simulink model "Flex_simulink"  (R2018a)
settings: Solver=FixedStepDiscrete  StartTime=0.0  StopTime=inf  FixedStep=0.00005  RelTol=1e-3  EnableMultiTasking=on
PreLoadFcn:
  | Ts = 0.001;
InitFcn:
  | Ts = 0.001;
values from neighbouring files (symbols this model uses):
  I_limit = 500    [init.m]
libraries: xpcethercatlib x91, simulink x54, slrtlib x2
(part 2 of 2)

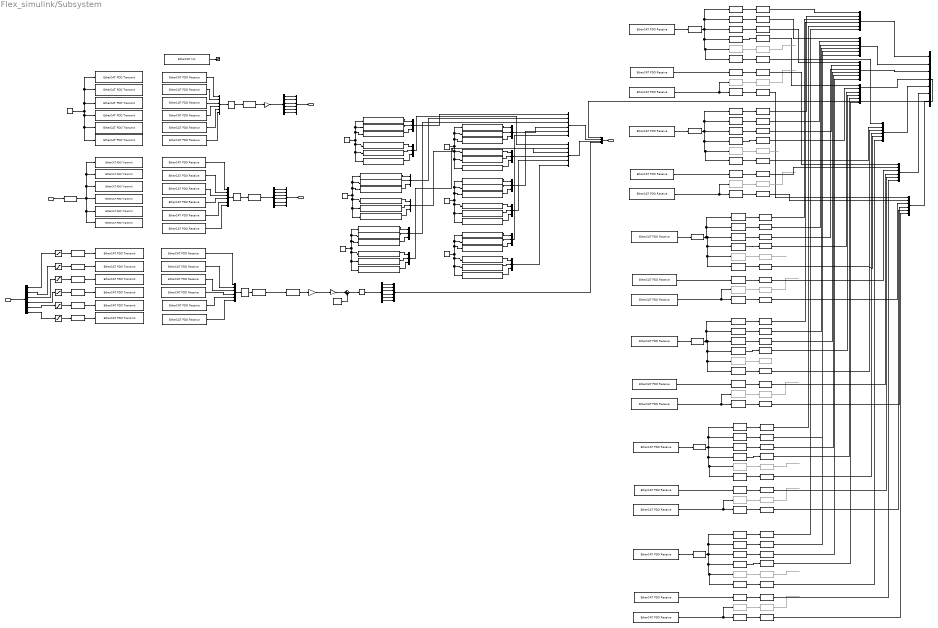
== system Flex_simulink/Subsystem ==
  Current [mA] : Inport
  Control word : Inport  Port=2
  Analog output voltage : Constant  Value=10000  OutDataTypeStr=int16
  Bus Creator{,2,4..8,20..21,23..28} (15 alike) : BusCreator  Inputs=6
  Bus Creator{1,3,10..19} (12 alike) : BusCreator  Inputs=3
  Bus Creator22 : BusCreator  Inputs=7
  Bus Creator9 : BusCreator  Inputs=4
  Bus Selector : BusSelector  OutputSignals=signal1,signal2,signal3,signal4,signal5,signal6
  Bus to Vector : BusToVector
  Bus to Vector1 : BusToVector
  Bus to Vector2 : BusToVector
  Constant : Constant  Value=-225
  Constant{1..6} (6 alike) : Constant  OutDataTypeStr=int32  SampleTime=1
  Data Type Conversion : DataTypeConversion  OutDataTypeStr=double
  Data Type Conversion1 : DataTypeConversion  OutDataTypeStr=double
  Data Type Conversion{3,10,21,27,31,37,41,47,51,57,61,67} (12 alike) : DataTypeConversion  Commented=on  OutDataTypeStr=boolean
  Data Type Conversion{2,6,8,11..14,22..26,28,30,32..36,38,40,42..46,48,50,52..56,58,60,62..66,68,70} (42 alike) : DataTypeConversion  OutDataTypeStr=boolean
  Data Type Conversion{4,9,15,17..20} (7 alike) : DataTypeConversion  OutDataTypeStr=int32
  Data Type Conversion16 : DataTypeConversion  OutDataTypeStr=uint16
  Data Type Conversion{7,29,39,49,59,69} (6 alike) : DataTypeConversion  OutDataTypeStr=uint16  RndMeth=Round
  Data Type Conversion5 : DataTypeConversion  OutDataTypeStr=double
  Demux : Demux  Outputs=6
  Demux1 : Demux  Outputs=6
  Demux2 : Demux  Outputs=6
  EtherCAT Async SDO Upload : xpcethercatlib/EtherCAT Async SDO Upload  index=8192  subIndex=1  sig_type=uint32  sig_dim=1  device_id=0  slave_name=Drive 2 (AKD)  sample_time=1  slave_addr=1001  selected_slave=Term 1 (EK1100)  timeout=500  slave_found=1
      settings: SourceProductName=Simulink Real-Time  SourceProductBaseCode=XP
  EtherCAT Async SDO Upload1 : xpcethercatlib/EtherCAT Async SDO Upload  index=8192  subIndex=2  sig_type=uint32  sig_dim=1  device_id=0  slave_name=Drive 2 (AKD)  sample_time=1  slave_addr=1001  selected_slave=Term 1 (EK1100)  timeout=500  slave_found=1
      settings: SourceProductName=Simulink Real-Time  SourceProductBaseCode=XP
  EtherCAT Async SDO Upload10 : xpcethercatlib/EtherCAT Async SDO Upload  index=8193  subIndex=2  sig_type=uint32  sig_dim=1  device_id=0  slave_name=Drive 3 (AKD)  sample_time=1  slave_addr=1002  selected_slave=Term 1 (EK1100)  timeout=500  slave_found=1
      settings: SourceProductName=Simulink Real-Time  SourceProductBaseCode=XP
  EtherCAT Async SDO Upload11 : xpcethercatlib/EtherCAT Async SDO Upload  index=8193  subIndex=3  sig_type=uint32  sig_dim=1  device_id=0  slave_name=Drive 3 (AKD)  sample_time=1  slave_addr=1002  selected_slave=Term 1 (EK1100)  timeout=500  slave_found=1
      settings: SourceProductName=Simulink Real-Time  SourceProductBaseCode=XP
  EtherCAT Async SDO Upload12 : xpcethercatlib/EtherCAT Async SDO Upload  index=8192  subIndex=1  sig_type=uint32  sig_dim=1  device_id=0  slave_name=Drive 4 (AKD)  sample_time=1  slave_addr=1003  selected_slave=Term 1 (EK1100)  timeout=500  slave_found=1
      settings: SourceProductName=Simulink Real-Time  SourceProductBaseCode=XP
  EtherCAT Async SDO Upload13 : xpcethercatlib/EtherCAT Async SDO Upload  index=8192  subIndex=2  sig_type=uint32  sig_dim=1  device_id=0  slave_name=Drive 4 (AKD)  sample_time=1  slave_addr=1003  selected_slave=Term 1 (EK1100)  timeout=500  slave_found=1
      settings: SourceProductName=Simulink Real-Time  SourceProductBaseCode=XP
  EtherCAT Async SDO Upload14 : xpcethercatlib/EtherCAT Async SDO Upload  index=8192  subIndex=3  sig_type=uint32  sig_dim=1  device_id=0  slave_name=Drive 4 (AKD)  sample_time=1  slave_addr=1003  selected_slave=Term 1 (EK1100)  timeout=500  slave_found=1
      settings: SourceProductName=Simulink Real-Time  SourceProductBaseCode=XP
  EtherCAT Async SDO Upload15 : xpcethercatlib/EtherCAT Async SDO Upload  index=8193  subIndex=1  sig_type=uint32  sig_dim=1  device_id=0  slave_name=Drive 4 (AKD)  sample_time=1  slave_addr=1003  selected_slave=Term 1 (EK1100)  timeout=500  slave_found=1
      settings: SourceProductName=Simulink Real-Time  SourceProductBaseCode=XP
  EtherCAT Async SDO Upload16 : xpcethercatlib/EtherCAT Async SDO Upload  index=8193  subIndex=2  sig_type=uint32  sig_dim=1  device_id=0  slave_name=Drive 4 (AKD)  sample_time=1  slave_addr=1003  selected_slave=Term 1 (EK1100)  timeout=500  slave_found=1
      settings: SourceProductName=Simulink Real-Time  SourceProductBaseCode=XP
  EtherCAT Async SDO Upload17 : xpcethercatlib/EtherCAT Async SDO Upload  index=8193  subIndex=3  sig_type=uint32  sig_dim=1  device_id=0  slave_name=Drive 4 (AKD)  sample_time=1  slave_addr=1003  selected_slave=Term 1 (EK1100)  timeout=500  slave_found=1
      settings: SourceProductName=Simulink Real-Time  SourceProductBaseCode=XP
  EtherCAT Async SDO Upload18 : xpcethercatlib/EtherCAT Async SDO Upload  index=8192  subIndex=1  sig_type=uint32  sig_dim=1  device_id=0  slave_name=Drive 5 (AKD)  sample_time=1  slave_addr=1004  selected_slave=Term 1 (EK1100)  timeout=500  slave_found=1
      settings: SourceProductName=Simulink Real-Time  SourceProductBaseCode=XP
  EtherCAT Async SDO Upload19 : xpcethercatlib/EtherCAT Async SDO Upload  index=8192  subIndex=2  sig_type=uint32  sig_dim=1  device_id=0  slave_name=Drive 5 (AKD)  sample_time=1  slave_addr=1004  selected_slave=Term 1 (EK1100)  timeout=500  slave_found=1
      settings: SourceProductName=Simulink Real-Time  SourceProductBaseCode=XP
  EtherCAT Async SDO Upload2 : xpcethercatlib/EtherCAT Async SDO Upload  index=8192  subIndex=3  sig_type=uint32  sig_dim=1  device_id=0  slave_name=Drive 1 (AKD)  sample_time=1  slave_addr=1001  selected_slave=Term 1 (EK1100)  timeout=500  slave_found=1
      settings: SourceProductName=Simulink Real-Time  SourceProductBaseCode=XP
  EtherCAT Async SDO Upload20 : xpcethercatlib/EtherCAT Async SDO Upload  index=8192  subIndex=3  sig_type=uint32  sig_dim=1  device_id=0  slave_name=Drive 5 (AKD)  sample_time=1  slave_addr=1004  selected_slave=Term 1 (EK1100)  timeout=500  slave_found=1
      settings: SourceProductName=Simulink Real-Time  SourceProductBaseCode=XP
  EtherCAT Async SDO Upload21 : xpcethercatlib/EtherCAT Async SDO Upload  index=8193  subIndex=1  sig_type=uint32  sig_dim=1  device_id=0  slave_name=Drive 5 (AKD)  sample_time=1  slave_addr=1004  selected_slave=Term 1 (EK1100)  timeout=500  slave_found=1
      settings: SourceProductName=Simulink Real-Time  SourceProductBaseCode=XP
  EtherCAT Async SDO Upload22 : xpcethercatlib/EtherCAT Async SDO Upload  index=8193  subIndex=2  sig_type=uint32  sig_dim=1  device_id=0  slave_name=Drive 5 (AKD)  sample_time=1  slave_addr=1004  selected_slave=Term 1 (EK1100)  timeout=500  slave_found=1
      settings: SourceProductName=Simulink Real-Time  SourceProductBaseCode=XP
  EtherCAT Async SDO Upload23 : xpcethercatlib/EtherCAT Async SDO Upload  index=8193  subIndex=3  sig_type=uint32  sig_dim=1  device_id=0  slave_name=Drive 5 (AKD)  sample_time=1  slave_addr=1004  selected_slave=Term 1 (EK1100)  timeout=500  slave_found=1
      settings: SourceProductName=Simulink Real-Time  SourceProductBaseCode=XP
  EtherCAT Async SDO Upload24 : xpcethercatlib/EtherCAT Async SDO Upload  index=8192  subIndex=1  sig_type=uint32  sig_dim=1  device_id=0  slave_name=Drive 6 (AKD)  sample_time=1  slave_addr=1005  selected_slave=Term 1 (EK1100)  timeout=500  slave_found=1
      settings: SourceProductName=Simulink Real-Time  SourceProductBaseCode=XP
  EtherCAT Async SDO Upload25 : xpcethercatlib/EtherCAT Async SDO Upload  index=8192  subIndex=2  sig_type=uint32  sig_dim=1  device_id=0  slave_name=Drive 6 (AKD)  sample_time=1  slave_addr=1005  selected_slave=Term 1 (EK1100)  timeout=500  slave_found=1
      settings: SourceProductName=Simulink Real-Time  SourceProductBaseCode=XP
  EtherCAT Async SDO Upload26 : xpcethercatlib/EtherCAT Async SDO Upload  index=8192  subIndex=3  sig_type=uint32  sig_dim=1  device_id=0  slave_name=Drive 6 (AKD)  sample_time=1  slave_addr=1005  selected_slave=Term 1 (EK1100)  timeout=500  slave_found=1
      settings: SourceProductName=Simulink Real-Time  SourceProductBaseCode=XP
  EtherCAT Async SDO Upload27 : xpcethercatlib/EtherCAT Async SDO Upload  index=8193  subIndex=1  sig_type=uint32  sig_dim=1  device_id=0  slave_name=Drive 6 (AKD)  sample_time=1  slave_addr=1005  selected_slave=Term 1 (EK1100)  timeout=500  slave_found=1
      settings: SourceProductName=Simulink Real-Time  SourceProductBaseCode=XP
  EtherCAT Async SDO Upload28 : xpcethercatlib/EtherCAT Async SDO Upload  index=8193  subIndex=2  sig_type=uint32  sig_dim=1  device_id=0  slave_name=Drive 6 (AKD)  sample_time=1  slave_addr=1005  selected_slave=Term 1 (EK1100)  timeout=500  slave_found=1
      settings: SourceProductName=Simulink Real-Time  SourceProductBaseCode=XP
  EtherCAT Async SDO Upload29 : xpcethercatlib/EtherCAT Async SDO Upload  index=8193  subIndex=3  sig_type=uint32  sig_dim=1  device_id=0  slave_name=Drive 6 (AKD)  sample_time=1  slave_addr=1005  selected_slave=Term 1 (EK1100)  timeout=500  slave_found=1
      settings: SourceProductName=Simulink Real-Time  SourceProductBaseCode=XP
  EtherCAT Async SDO Upload3 : xpcethercatlib/EtherCAT Async SDO Upload  index=8193  subIndex=1  sig_type=uint32  sig_dim=1  device_id=0  slave_name=Drive 1 (AKD)  sample_time=1  slave_addr=1001  selected_slave=Term 1 (EK1100)  timeout=500  slave_found=1
      settings: SourceProductName=Simulink Real-Time  SourceProductBaseCode=XP
  EtherCAT Async SDO Upload30 : xpcethercatlib/EtherCAT Async SDO Upload  index=8192  subIndex=1  sig_type=uint32  sig_dim=1  device_id=0  slave_name=Drive 7 (AKD)  sample_time=1  slave_addr=1006  selected_slave=Term 1 (EK1100)  timeout=500  slave_found=1
      settings: SourceProductName=Simulink Real-Time  SourceProductBaseCode=XP
  EtherCAT Async SDO Upload31 : xpcethercatlib/EtherCAT Async SDO Upload  index=8192  subIndex=2  sig_type=uint32  sig_dim=1  device_id=0  slave_name=Drive 7 (AKD)  sample_time=1  slave_addr=1006  selected_slave=Term 1 (EK1100)  timeout=500  slave_found=1
      settings: SourceProductName=Simulink Real-Time  SourceProductBaseCode=XP
  EtherCAT Async SDO Upload32 : xpcethercatlib/EtherCAT Async SDO Upload  index=8192  subIndex=3  sig_type=uint32  sig_dim=1  device_id=0  slave_name=Drive 7 (AKD)  sample_time=1  slave_addr=1006  selected_slave=Term 1 (EK1100)  timeout=500  slave_found=1
      settings: SourceProductName=Simulink Real-Time  SourceProductBaseCode=XP
  EtherCAT Async SDO Upload33 : xpcethercatlib/EtherCAT Async SDO Upload  index=8193  subIndex=1  sig_type=uint32  sig_dim=1  device_id=0  slave_name=Drive 7 (AKD)  sample_time=1  slave_addr=1006  selected_slave=Term 1 (EK1100)  timeout=500  slave_found=1
      settings: SourceProductName=Simulink Real-Time  SourceProductBaseCode=XP
  EtherCAT Async SDO Upload34 : xpcethercatlib/EtherCAT Async SDO Upload  index=8193  subIndex=2  sig_type=uint32  sig_dim=1  device_id=0  slave_name=Drive 7 (AKD)  sample_time=1  slave_addr=1006  selected_slave=Term 1 (EK1100)  timeout=500  slave_found=1
      settings: SourceProductName=Simulink Real-Time  SourceProductBaseCode=XP
  EtherCAT Async SDO Upload35 : xpcethercatlib/EtherCAT Async SDO Upload  index=8193  subIndex=3  sig_type=uint32  sig_dim=1  device_id=0  slave_name=Drive 7 (AKD)  sample_time=1  slave_addr=1006  selected_slave=Term 1 (EK1100)  timeout=500  slave_found=1
      settings: SourceProductName=Simulink Real-Time  SourceProductBaseCode=XP
  EtherCAT Async SDO Upload4 : xpcethercatlib/EtherCAT Async SDO Upload  index=8193  subIndex=2  sig_type=uint32  sig_dim=1  device_id=0  slave_name=Drive 2 (AKD)  sample_time=1  slave_addr=1001  selected_slave=Term 1 (EK1100)  timeout=500  slave_found=1
      settings: SourceProductName=Simulink Real-Time  SourceProductBaseCode=XP
  EtherCAT Async SDO Upload5 : xpcethercatlib/EtherCAT Async SDO Upload  index=8193  subIndex=3  sig_type=uint32  sig_dim=1  device_id=0  slave_name=Drive 1 (AKD)  sample_time=1  slave_addr=1001  selected_slave=Term 1 (EK1100)  timeout=500  slave_found=1
      settings: SourceProductName=Simulink Real-Time  SourceProductBaseCode=XP
  EtherCAT Async SDO Upload6 : xpcethercatlib/EtherCAT Async SDO Upload  index=8192  subIndex=1  sig_type=uint32  sig_dim=1  device_id=0  slave_name=Drive 3 (AKD)  sample_time=1  slave_addr=1002  selected_slave=Term 1 (EK1100)  timeout=500  slave_found=1
      settings: SourceProductName=Simulink Real-Time  SourceProductBaseCode=XP
  EtherCAT Async SDO Upload7 : xpcethercatlib/EtherCAT Async SDO Upload  index=8192  subIndex=2  sig_type=uint32  sig_dim=1  device_id=0  slave_name=Drive 3 (AKD)  sample_time=1  slave_addr=1002  selected_slave=Term 1 (EK1100)  timeout=500  slave_found=1
      settings: SourceProductName=Simulink Real-Time  SourceProductBaseCode=XP
  EtherCAT Async SDO Upload8 : xpcethercatlib/EtherCAT Async SDO Upload  index=8192  subIndex=3  sig_type=uint32  sig_dim=1  device_id=0  slave_name=Drive 3 (AKD)  sample_time=1  slave_addr=1002  selected_slave=Term 1 (EK1100)  timeout=500  slave_found=1
      settings: SourceProductName=Simulink Real-Time  SourceProductBaseCode=XP
  EtherCAT Async SDO Upload9 : xpcethercatlib/EtherCAT Async SDO Upload  index=8193  subIndex=1  sig_type=uint32  sig_dim=1  device_id=0  slave_name=Drive 3 (AKD)  sample_time=1  slave_addr=1002  selected_slave=Term 1 (EK1100)  timeout=500  slave_found=1
      settings: SourceProductName=Simulink Real-Time  SourceProductBaseCode=XP
  "EtherCAT Init " : xpcethercatlib/EtherCAT Init   Priority=0  config_file=C:\Users\Mark\Desktop\tflex\sandbox_6drives\pdo_mapping_6dr.xml  device_id=0  pci_bus=13  pci_slot=0  pci_function=0  dctuning=0  enaDebug=off  enaDC=on  errLink=off  masterDbg=off  stateChgDbg=off  baseClock=off  masterCfg=off  logFile='c:\dbglog.txt'  sample_time=0.000250  DCMode=2
      settings: SourceProductName=Simulink Real-Time  SourceProductBaseCode=XP
  EtherCAT PDO Receive : xpcethercatlib/EtherCAT PDO Receive  Priority=2  sig_name=Drive 2 (AKD).Inputs_1.Position actual internal value  sig_offset=560  sig_type=int32  type_size=32  sig_dim=1  device_id=0  sample_time=0.000250
      settings: SourceProductName=Simulink Real-Time  SourceProductBaseCode=XP
  EtherCAT PDO Receive1 : xpcethercatlib/EtherCAT PDO Receive  Priority=2  sig_name=Drive 2 (AKD).Inputs.AOUT_INPUT_VALUE  sig_offset=480  sig_type=int16  type_size=16  sig_dim=1  device_id=0  sample_time=0.000250
      settings: SourceProductName=Simulink Real-Time  SourceProductBaseCode=XP
  EtherCAT PDO Receive10 : xpcethercatlib/EtherCAT PDO Receive  Priority=2  sig_name=Drive 7 (AKD).Inputs_1.Position actual internal value  sig_offset=37488  sig_type=int32  type_size=32  sig_dim=1  device_id=0  sample_time=0.000250
      settings: SourceProductName=Simulink Real-Time  SourceProductBaseCode=XP
  EtherCAT PDO Receive11 : xpcethercatlib/EtherCAT PDO Receive  Priority=2  sig_name=Drive 3 (AKD).Inputs_1.Current actual value  sig_offset=12560  sig_type=int32  type_size=32  sig_dim=1  device_id=0  sample_time=0.000250
      settings: SourceProductName=Simulink Real-Time  SourceProductBaseCode=XP
  EtherCAT PDO Receive12 : xpcethercatlib/EtherCAT PDO Receive  Priority=2  sig_name=Drive 4 (AKD).Inputs_1.Current actual value  sig_offset=24848  sig_type=int32  type_size=32  sig_dim=1  device_id=0  sample_time=0.000250
      settings: SourceProductName=Simulink Real-Time  SourceProductBaseCode=XP
  EtherCAT PDO Receive13 : xpcethercatlib/EtherCAT PDO Receive  Priority=2  sig_name=Drive 5 (AKD).Inputs_1.Current actual value  sig_offset=37136  sig_type=int32  type_size=32  sig_dim=1  device_id=0  sample_time=0.000250
      settings: SourceProductName=Simulink Real-Time  SourceProductBaseCode=XP
  EtherCAT PDO Receive14 : xpcethercatlib/EtherCAT PDO Receive  Priority=2  sig_name=Drive 6 (AKD).Inputs_1.Current actual value  sig_offset=37296  sig_type=int32  type_size=32  sig_dim=1  device_id=0  sample_time=0.000250
      settings: SourceProductName=Simulink Real-Time  SourceProductBaseCode=XP
  EtherCAT PDO Receive15 : xpcethercatlib/EtherCAT PDO Receive  Priority=2  sig_name=Drive 7 (AKD).Inputs_1.Current actual value  sig_offset=37456  sig_type=int32  type_size=32  sig_dim=1  device_id=0  sample_time=0.000250
      settings: SourceProductName=Simulink Real-Time  SourceProductBaseCode=XP
  EtherCAT PDO Receive16 : xpcethercatlib/EtherCAT PDO Receive  Priority=2  sig_name=Drive 3 (AKD).Inputs.AOUT_INPUT_VALUE  sig_offset=12512  sig_type=int16  type_size=16  sig_dim=1  device_id=0  sample_time=0.000250
      settings: SourceProductName=Simulink Real-Time  SourceProductBaseCode=XP
  EtherCAT PDO Receive17 : xpcethercatlib/EtherCAT PDO Receive  Priority=2  sig_name=Drive 4 (AKD).Inputs.AOUT_INPUT_VALUE  sig_offset=24800  sig_type=int16  type_size=16  sig_dim=1  device_id=0  sample_time=0.000250
      settings: SourceProductName=Simulink Real-Time  SourceProductBaseCode=XP
  EtherCAT PDO Receive18 : xpcethercatlib/EtherCAT PDO Receive  Priority=2  sig_name=Drive 5 (AKD).Inputs.AOUT_INPUT_VALUE  sig_offset=37088  sig_type=int16  type_size=16  sig_dim=1  device_id=0  sample_time=0.000250
      settings: SourceProductName=Simulink Real-Time  SourceProductBaseCode=XP
  EtherCAT PDO Receive19 : xpcethercatlib/EtherCAT PDO Receive  Priority=2  sig_name=Drive 6 (AKD).Inputs.AOUT_INPUT_VALUE  sig_offset=37248  sig_type=int16  type_size=16  sig_dim=1  device_id=0  sample_time=0.000250
      settings: SourceProductName=Simulink Real-Time  SourceProductBaseCode=XP
  EtherCAT PDO Receive2 : xpcethercatlib/EtherCAT PDO Receive  Priority=2  sig_name=Drive 2 (AKD).Inputs_1.Current actual value  sig_offset=528  sig_type=int32  type_size=32  sig_dim=1  device_id=0  sample_time=0.000250
      settings: SourceProductName=Simulink Real-Time  SourceProductBaseCode=XP
  EtherCAT PDO Receive20 : xpcethercatlib/EtherCAT PDO Receive  Priority=2  sig_name=Drive 7 (AKD).Inputs.AOUT_INPUT_VALUE  sig_offset=37408  sig_type=int16  type_size=16  sig_dim=1  device_id=0  sample_time=0.000250
      settings: SourceProductName=Simulink Real-Time  SourceProductBaseCode=XP
  EtherCAT PDO Receive21 : xpcethercatlib/EtherCAT PDO Receive  Priority=2  sig_name=Drive 3 (AKD).Inputs.Digital inputs  sig_offset=12528  sig_type=uint32  type_size=32  sig_dim=1  device_id=0  sample_time=0.000250
      settings: SourceProductName=Simulink Real-Time  SourceProductBaseCode=XP
  EtherCAT PDO Receive22 : xpcethercatlib/EtherCAT PDO Receive  Priority=2  sig_name=Drive 3 (AKD).Inputs.Statusword  sig_offset=12496  sig_type=uint16  type_size=16  sig_dim=1  device_id=0  sample_time=0.000250
      settings: SourceProductName=Simulink Real-Time  SourceProductBaseCode=XP
  EtherCAT PDO Receive23 : xpcethercatlib/EtherCAT PDO Receive  Priority=2  sig_name=Drive 3 (AKD).Inputs_2.Manufacturer status register  sig_offset=12624  sig_type=uint32  type_size=32  sig_dim=1  device_id=0  sample_time=0.000250
      settings: SourceProductName=Simulink Real-Time  SourceProductBaseCode=XP
  EtherCAT PDO Receive24 : xpcethercatlib/EtherCAT PDO Receive  Priority=2  sig_name=Drive 4 (AKD).Inputs.Digital inputs  sig_offset=24816  sig_type=uint32  type_size=32  sig_dim=1  device_id=0  sample_time=0.000250
      settings: SourceProductName=Simulink Real-Time  SourceProductBaseCode=XP
  EtherCAT PDO Receive25 : xpcethercatlib/EtherCAT PDO Receive  Priority=2  sig_name=Drive 4 (AKD).Inputs.Statusword  sig_offset=24784  sig_type=uint16  type_size=16  sig_dim=1  device_id=0  sample_time=0.000250
      settings: SourceProductName=Simulink Real-Time  SourceProductBaseCode=XP
  EtherCAT PDO Receive26 : xpcethercatlib/EtherCAT PDO Receive  Priority=2  sig_name=Drive 4 (AKD).Inputs_2.Manufacturer status register  sig_offset=24912  sig_type=uint32  type_size=32  sig_dim=1  device_id=0  sample_time=0.000250
      settings: SourceProductName=Simulink Real-Time  SourceProductBaseCode=XP
  EtherCAT PDO Receive27 : xpcethercatlib/EtherCAT PDO Receive  Priority=2  sig_name=Drive 5 (AKD).Inputs.Digital inputs  sig_offset=37104  sig_type=uint32  type_size=32  sig_dim=1  device_id=0  sample_time=0.000250
      settings: SourceProductName=Simulink Real-Time  SourceProductBaseCode=XP
  EtherCAT PDO Receive28 : xpcethercatlib/EtherCAT PDO Receive  Priority=2  sig_name=Drive 5 (AKD).Inputs.Statusword  sig_offset=37072  sig_type=uint16  type_size=16  sig_dim=1  device_id=0  sample_time=0.000250
      settings: SourceProductName=Simulink Real-Time  SourceProductBaseCode=XP
  EtherCAT PDO Receive29 : xpcethercatlib/EtherCAT PDO Receive  Priority=2  sig_name=Drive 5 (AKD).Inputs_2.Manufacturer status register  sig_offset=37200  sig_type=uint32  type_size=32  sig_dim=1  device_id=0  sample_time=0.000250
      settings: SourceProductName=Simulink Real-Time  SourceProductBaseCode=XP
  EtherCAT PDO Receive3 : xpcethercatlib/EtherCAT PDO Receive  Priority=2  sig_name=Drive 2 (AKD).Inputs.Digital inputs  sig_offset=496  sig_type=uint32  type_size=32  sig_dim=1  device_id=0  sample_time=0.000250
      settings: SourceProductName=Simulink Real-Time  SourceProductBaseCode=XP
  EtherCAT PDO Receive30 : xpcethercatlib/EtherCAT PDO Receive  Priority=2  sig_name=Drive 6 (AKD).Inputs.Digital inputs  sig_offset=37264  sig_type=uint32  type_size=32  sig_dim=1  device_id=0  sample_time=0.000250
      settings: SourceProductName=Simulink Real-Time  SourceProductBaseCode=XP
  EtherCAT PDO Receive31 : xpcethercatlib/EtherCAT PDO Receive  Priority=2  sig_name=Drive 6 (AKD).Inputs.Statusword  sig_offset=37232  sig_type=uint16  type_size=16  sig_dim=1  device_id=0  sample_time=0.000250
      settings: SourceProductName=Simulink Real-Time  SourceProductBaseCode=XP
  EtherCAT PDO Receive32 : xpcethercatlib/EtherCAT PDO Receive  Priority=2  sig_name=Drive 6 (AKD).Inputs_2.Manufacturer status register  sig_offset=37360  sig_type=uint32  type_size=32  sig_dim=1  device_id=0  sample_time=0.000250
      settings: SourceProductName=Simulink Real-Time  SourceProductBaseCode=XP
  EtherCAT PDO Receive33 : xpcethercatlib/EtherCAT PDO Receive  Priority=2  sig_name=Drive 7 (AKD).Inputs.Digital inputs  sig_offset=37424  sig_type=uint32  type_size=32  sig_dim=1  device_id=0  sample_time=0.000250
      settings: SourceProductName=Simulink Real-Time  SourceProductBaseCode=XP
  EtherCAT PDO Receive34 : xpcethercatlib/EtherCAT PDO Receive  Priority=2  sig_name=Drive 7 (AKD).Inputs.Statusword  sig_offset=37392  sig_type=uint16  type_size=16  sig_dim=1  device_id=0  sample_time=0.000250
      settings: SourceProductName=Simulink Real-Time  SourceProductBaseCode=XP
  EtherCAT PDO Receive35 : xpcethercatlib/EtherCAT PDO Receive  Priority=2  sig_name=Drive 7 (AKD).Inputs_2.Manufacturer status register  sig_offset=37520  sig_type=uint32  type_size=32  sig_dim=1  device_id=0  sample_time=0.000250
      settings: SourceProductName=Simulink Real-Time  SourceProductBaseCode=XP
  EtherCAT PDO Receive4 : xpcethercatlib/EtherCAT PDO Receive  Priority=2  sig_name=Drive 2 (AKD).Inputs.Statusword  sig_offset=464  sig_type=uint16  type_size=16  sig_dim=1  device_id=0  sample_time=0.000250
      settings: SourceProductName=Simulink Real-Time  SourceProductBaseCode=XP
  EtherCAT PDO Receive5 : xpcethercatlib/EtherCAT PDO Receive  Priority=2  sig_name=Drive 2 (AKD).Inputs_2.Manufacturer status register  sig_offset=592  sig_type=uint32  type_size=32  sig_dim=1  device_id=0  sample_time=0.000250
      settings: SourceProductName=Simulink Real-Time  SourceProductBaseCode=XP
  EtherCAT PDO Receive6 : xpcethercatlib/EtherCAT PDO Receive  Priority=2  sig_name=Drive 3 (AKD).Inputs_1.Position actual internal value  sig_offset=12592  sig_type=int32  type_size=32  sig_dim=1  device_id=0  sample_time=0.000250
      settings: SourceProductName=Simulink Real-Time  SourceProductBaseCode=XP
  EtherCAT PDO Receive7 : xpcethercatlib/EtherCAT PDO Receive  Priority=2  sig_name=Drive 4 (AKD).Inputs_1.Position actual internal value  sig_offset=24880  sig_type=int32  type_size=32  sig_dim=1  device_id=0  sample_time=0.000250
      settings: SourceProductName=Simulink Real-Time  SourceProductBaseCode=XP
  EtherCAT PDO Receive8 : xpcethercatlib/EtherCAT PDO Receive  Priority=2  sig_name=Drive 5 (AKD).Inputs_1.Position actual internal value  sig_offset=37168  sig_type=int32  type_size=32  sig_dim=1  device_id=0  sample_time=0.000250
      settings: SourceProductName=Simulink Real-Time  SourceProductBaseCode=XP
  EtherCAT PDO Receive9 : xpcethercatlib/EtherCAT PDO Receive  Priority=2  sig_name=Drive 6 (AKD).Inputs_1.Position actual internal value  sig_offset=37328  sig_type=int32  type_size=32  sig_dim=1  device_id=0  sample_time=0.000250
      settings: SourceProductName=Simulink Real-Time  SourceProductBaseCode=XP
  "EtherCAT PDO Transmit " : xpcethercatlib/EtherCAT PDO Transmit   Priority=3  sig_name=Drive 2 (AKD).Outputs.AOUT.VALUE write  sig_offset=480  sig_type=int16  type_size=16  sig_dim=1  device_id=0  sample_time=0.000250
      settings: SourceProductName=Simulink Real-Time  SourceProductBaseCode=XP
  EtherCAT PDO Transmit 1 : xpcethercatlib/EtherCAT PDO Transmit   Priority=3  sig_name=Drive 2 (AKD).Outputs.Controlword  sig_offset=464  sig_type=uint16  type_size=16  sig_dim=1  device_id=0  sample_time=0.000250
      settings: SourceProductName=Simulink Real-Time  SourceProductBaseCode=XP
  EtherCAT PDO Transmit 10 : xpcethercatlib/EtherCAT PDO Transmit   Priority=3  sig_name=Drive 5 (AKD).Outputs.Controlword  sig_offset=37072  sig_type=uint16  type_size=16  sig_dim=1  device_id=0  sample_time=0.000250
      settings: SourceProductName=Simulink Real-Time  SourceProductBaseCode=XP
  EtherCAT PDO Transmit 11 : xpcethercatlib/EtherCAT PDO Transmit   Priority=3  sig_name=Drive 6 (AKD).Outputs.Controlword  sig_offset=37232  sig_type=uint16  type_size=16  sig_dim=1  device_id=0  sample_time=0.000250
      settings: SourceProductName=Simulink Real-Time  SourceProductBaseCode=XP
  EtherCAT PDO Transmit 12 : xpcethercatlib/EtherCAT PDO Transmit   Priority=3  sig_name=Drive 7 (AKD).Outputs.Controlword  sig_offset=37392  sig_type=uint16  type_size=16  sig_dim=1  device_id=0  sample_time=0.000250
      settings: SourceProductName=Simulink Real-Time  SourceProductBaseCode=XP
  EtherCAT PDO Transmit 13 : xpcethercatlib/EtherCAT PDO Transmit   Priority=3  sig_name=Drive 3 (AKD).Outputs.Target current  sig_offset=12528  sig_type=int32  type_size=32  sig_dim=1  device_id=0  sample_time=0.000250
      settings: SourceProductName=Simulink Real-Time  SourceProductBaseCode=XP
  EtherCAT PDO Transmit 14 : xpcethercatlib/EtherCAT PDO Transmit   Priority=3  sig_name=Drive 4 (AKD).Outputs.Target current  sig_offset=24816  sig_type=int32  type_size=32  sig_dim=1  device_id=0  sample_time=0.000250
      settings: SourceProductName=Simulink Real-Time  SourceProductBaseCode=XP
  EtherCAT PDO Transmit 15 : xpcethercatlib/EtherCAT PDO Transmit   Priority=3  sig_name=Drive 5 (AKD).Outputs.Target current  sig_offset=37104  sig_type=int32  type_size=32  sig_dim=1  device_id=0  sample_time=0.000250
      settings: SourceProductName=Simulink Real-Time  SourceProductBaseCode=XP
  EtherCAT PDO Transmit 16 : xpcethercatlib/EtherCAT PDO Transmit   Priority=3  sig_name=Drive 6 (AKD).Outputs.Target current  sig_offset=37264  sig_type=int32  type_size=32  sig_dim=1  device_id=0  sample_time=0.000250
      settings: SourceProductName=Simulink Real-Time  SourceProductBaseCode=XP
  EtherCAT PDO Transmit 17 : xpcethercatlib/EtherCAT PDO Transmit   Priority=3  sig_name=Drive 7 (AKD).Outputs.Target current  sig_offset=37424  sig_type=int32  type_size=32  sig_dim=1  device_id=0  sample_time=0.000250
      settings: SourceProductName=Simulink Real-Time  SourceProductBaseCode=XP
  EtherCAT PDO Transmit 2 : xpcethercatlib/EtherCAT PDO Transmit   Priority=3  sig_name=Drive 3 (AKD).Outputs.AOUT.VALUE write  sig_offset=12512  sig_type=int16  type_size=16  sig_dim=1  device_id=0  sample_time=0.000250
      settings: SourceProductName=Simulink Real-Time  SourceProductBaseCode=XP
  EtherCAT PDO Transmit 3 : xpcethercatlib/EtherCAT PDO Transmit   Priority=3  sig_name=Drive 2 (AKD).Outputs.Target current  sig_offset=496  sig_type=int32  type_size=32  sig_dim=1  device_id=0  sample_time=0.000250
      settings: SourceProductName=Simulink Real-Time  SourceProductBaseCode=XP
  EtherCAT PDO Transmit 4 : xpcethercatlib/EtherCAT PDO Transmit   Priority=3  sig_name=Drive 4 (AKD).Outputs.AOUT.VALUE write  sig_offset=24800  sig_type=int16  type_size=16  sig_dim=1  device_id=0  sample_time=0.000250
      settings: SourceProductName=Simulink Real-Time  SourceProductBaseCode=XP
  EtherCAT PDO Transmit 5 : xpcethercatlib/EtherCAT PDO Transmit   Priority=3  sig_name=Drive 5 (AKD).Outputs.AOUT.VALUE write  sig_offset=37088  sig_type=int16  type_size=16  sig_dim=1  device_id=0  sample_time=0.000250
      settings: SourceProductName=Simulink Real-Time  SourceProductBaseCode=XP
  EtherCAT PDO Transmit 6 : xpcethercatlib/EtherCAT PDO Transmit   Priority=3  sig_name=Drive 6 (AKD).Outputs.AOUT.VALUE write  sig_offset=37248  sig_type=int16  type_size=16  sig_dim=1  device_id=0  sample_time=0.000250
      settings: SourceProductName=Simulink Real-Time  SourceProductBaseCode=XP
  EtherCAT PDO Transmit 7 : xpcethercatlib/EtherCAT PDO Transmit   Priority=3  sig_name=Drive 7 (AKD).Outputs.AOUT.VALUE write  sig_offset=37408  sig_type=int16  type_size=16  sig_dim=1  device_id=0  sample_time=0.000250
      settings: SourceProductName=Simulink Real-Time  SourceProductBaseCode=XP
  EtherCAT PDO Transmit 8 : xpcethercatlib/EtherCAT PDO Transmit   Priority=3  sig_name=Drive 3 (AKD).Outputs.Controlword  sig_offset=12496  sig_type=uint16  type_size=16  sig_dim=1  device_id=0  sample_time=0.000250
      settings: SourceProductName=Simulink Real-Time  SourceProductBaseCode=XP
  EtherCAT PDO Transmit 9 : xpcethercatlib/EtherCAT PDO Transmit   Priority=3  sig_name=Drive 4 (AKD).Outputs.Controlword  sig_offset=24784  sig_type=uint16  type_size=16  sig_dim=1  device_id=0  sample_time=0.000250
      settings: SourceProductName=Simulink Real-Time  SourceProductBaseCode=XP
  Extract Bits{,9,18,27,36,45} (6 alike) : simulink/Logic and Bit Operations/Extract Bits  bitsToExtract=Range of bits  numBits=8  bitIdxRange=[16]  outScalingMode=Treat bit field as an integer
      settings: SourceProductName=Simulink
  Extract Bits{1,10,19,28,37,46} (6 alike) : simulink/Logic and Bit Operations/Extract Bits  bitsToExtract=Range of bits  numBits=8  bitIdxRange=[0]  outScalingMode=Treat bit field as an integer
      settings: SourceProductName=Simulink
  Extract Bits{2,11,20,29,38,47} (6 alike) : simulink/Logic and Bit Operations/Extract Bits  bitsToExtract=Range of bits  numBits=8  bitIdxRange=[1]  outScalingMode=Treat bit field as an integer
      settings: SourceProductName=Simulink
  Extract Bits{3,12,21,30,39,48} (6 alike) : simulink/Logic and Bit Operations/Extract Bits  bitsToExtract=Range of bits  numBits=8  bitIdxRange=[2]  outScalingMode=Treat bit field as an integer
      settings: SourceProductName=Simulink
  Extract Bits{4,13,22,31,40,49} (6 alike) : simulink/Logic and Bit Operations/Extract Bits  bitsToExtract=Range of bits  numBits=8  bitIdxRange=[3]  outScalingMode=Treat bit field as an integer
      settings: SourceProductName=Simulink
  Extract Bits{5,14,23,32,41,50} (6 alike) : simulink/Logic and Bit Operations/Extract Bits  Commented=on  bitsToExtract=Range of bits  numBits=8  bitIdxRange=[5]  outScalingMode=Treat bit field as an integer
      settings: SourceProductName=Simulink
  Extract Bits{6,15,24,33,42,51} (6 alike) : simulink/Logic and Bit Operations/Extract Bits  bitsToExtract=Range of bits  numBits=8  bitIdxRange=[6]  outScalingMode=Treat bit field as an integer
      settings: SourceProductName=Simulink
  Extract Bits{7,16,25,34,43,52} (6 alike) : simulink/Logic and Bit Operations/Extract Bits  bitsToExtract=Range of bits  numBits=8  bitIdxRange=[13]  outScalingMode=Treat bit field as an integer
      settings: SourceProductName=Simulink
  Extract Bits{8,17,26,35,44,53} (6 alike) : simulink/Logic and Bit Operations/Extract Bits  Commented=on  bitsToExtract=Range of bits  numBits=8  bitIdxRange=[29]  outScalingMode=Treat bit field as an integer
      settings: SourceProductName=Simulink
  Gain : Gain  Gain=360/(2^32)
  Gain2 : Gain  Gain=12.5/(2^15-1)
  Gain3 : Gain  Gain=215
  Rounding Function : Rounding
  Saturation{,1..5} (6 alike) : Saturate  UpperLimit=I_limit  LowerLimit=-I_limit
  Sum1 : Sum  Inputs=|++  OutDataTypeStr=double
  Terminator : Terminator
  Angle [degrees] : Outport
  Actual current [mA] : Outport  Port=2
  Status : Outport  Port=3
  wires:
  Extract Bits3/1 -> Data Type Conversion12/1  "operation enable"
  EtherCAT Async SDO Upload4/1 -> Bus Creator3/2
  Data Type Conversion9/1 -> EtherCAT PDO Transmit 3/1  "Input current [mA]"
  Extract Bits7/1 -> Data Type Conversion2/1  "STO selected"
  EtherCAT PDO Receive2/1 -> Bus Creator4/1  "Actual Current [mA]"
  EtherCAT Async SDO Upload3/1 -> Bus Creator3/1
  Data Type Conversion14/1 -> Bus Creator2/1  "ready to switch on"
  Gain3/1 -> Sum1/1
  EtherCAT Async SDO Upload2/1 -> Bus Creator1/3
  EtherCAT PDO Receive1/1 -> Bus Creator5/1  "Analog input [bits]"
  Data Type Conversion5/1 -> Gain2/1
  EtherCAT Async SDO Upload/1 -> Bus Creator1/1
  Data Type Conversion11/1 -> Bus Creator25/1  "fault"
  Data Type Conversion3/1 -> ?  "HW enabled"
  Data Type Conversion8/1 -> Bus Creator27/1  "in limits"
  Data Type Conversion13/1 -> Bus Creator23/1  "switched on"
  Data Type Conversion7/1 -> Extract Bits1/1, Extract Bits2/1, Extract Bits3/1, Extract Bits4/1, Extract Bits6/1, Extract Bits5/1
  Data Type Conversion6/1 -> Bus Creator26/1  "switch on disable"
  Data Type Conversion/1 -> Gain/1
  EtherCAT PDO Receive5/1 -> Extract Bits8/1, Extract Bits7/1
  Data Type Conversion10/1 -> ?  "quick stop"
  Control word/1 -> Data Type Conversion16/1  "control word"
  Analog output voltage/1 -> EtherCAT PDO Transmit 7/1, EtherCAT PDO Transmit 6/1, EtherCAT PDO Transmit 5/1, EtherCAT PDO Transmit 4/1, EtherCAT PDO Transmit 2/1, "EtherCAT PDO Transmit "/1
  EtherCAT PDO Receive3/1 -> Extract Bits/1  "Digital inputs []"
  Current [mA]/1 -> Bus Selector/1  "Current [mA]"
  EtherCAT Async SDO Upload5/1 -> Bus Creator3/3
  Gain2/1 -> Gain3/1  "Analog in [V]"
  Extract Bits5/1 -> Data Type Conversion10/1  "quick stop"
  "EtherCAT Init "/1 -> Terminator/1
  EtherCAT Async SDO Upload1/1 -> Bus Creator1/2
  Extract Bits8/1 -> Data Type Conversion3/1
  Extract Bits1/1 -> Data Type Conversion14/1  "ready to switch on"
  Extract Bits/1 -> Data Type Conversion8/1  "limit  switch"
  Data Type Conversion16/1 -> EtherCAT PDO Transmit 12/1, EtherCAT PDO Transmit 11/1, EtherCAT PDO Transmit 10/1, EtherCAT PDO Transmit 9/1, EtherCAT PDO Transmit 8/1, EtherCAT PDO Transmit 1/1
  EtherCAT PDO Receive4/1 -> Data Type Conversion7/1
  Rounding Function/1 -> Demux2/1  "Temperature"
  Extract Bits4/1 -> Data Type Conversion11/1  "fault"
  Data Type Conversion2/1 -> Bus Creator28/1  "STO selected"
  Gain/1 -> Demux/1  "Angle [degrees]"
  Extract Bits2/1 -> Data Type Conversion13/1  "switched on"
  Extract Bits6/1 -> Data Type Conversion6/1  "switch on disable"
  Sum1/1 -> Rounding Function/1
  Constant1/1 -> EtherCAT Async SDO Upload2/1, EtherCAT Async SDO Upload1/1, EtherCAT Async SDO Upload/1, EtherCAT Async SDO Upload5/1, EtherCAT Async SDO Upload4/1, EtherCAT Async SDO Upload3/1
  Bus Creator3/1 -> Bus Creator21/1
  Constant/1 -> Sum1/2
  Bus Creator1/1 -> Bus Creator20/1
  Data Type Conversion4/1 -> Data Type Conversion5/1  "Analog input []"
  Data Type Conversion12/1 -> Bus Creator24/1  "operation enable"
  Saturation/1 -> Data Type Conversion9/1
  EtherCAT PDO Receive/1 -> Bus Creator/1
  EtherCAT PDO Receive6/1 -> Bus Creator/2
  EtherCAT PDO Receive7/1 -> Bus Creator/3
  EtherCAT PDO Receive8/1 -> Bus Creator/4
  EtherCAT PDO Receive9/1 -> Bus Creator/5
  EtherCAT PDO Receive10/1 -> Bus Creator/6
  Bus Creator/1 -> Bus to Vector/1
  Bus to Vector/1 -> Data Type Conversion/1
  EtherCAT PDO Receive11/1 -> Bus Creator4/2
  EtherCAT PDO Receive12/1 -> Bus Creator4/3
  EtherCAT PDO Receive13/1 -> Bus Creator4/4
  EtherCAT PDO Receive14/1 -> Bus Creator4/5
  EtherCAT PDO Receive15/1 -> Bus Creator4/6
  Bus Creator4/1 -> Bus to Vector1/1
  Bus to Vector1/1 -> Data Type Conversion1/1
  EtherCAT PDO Receive16/1 -> Bus Creator5/2
  EtherCAT PDO Receive17/1 -> Bus Creator5/3
  EtherCAT PDO Receive18/1 -> Bus Creator5/4
  EtherCAT PDO Receive19/1 -> Bus Creator5/5
  EtherCAT PDO Receive20/1 -> Bus Creator5/6
  Bus Creator5/1 -> Bus to Vector2/1
  Bus to Vector2/1 -> Data Type Conversion4/1
  Bus Selector/1 -> Saturation/1  "<signal1>"
  Data Type Conversion15/1 -> EtherCAT PDO Transmit 13/1  "Input current [mA]"
  Saturation1/1 -> Data Type Conversion15/1
  Data Type Conversion17/1 -> EtherCAT PDO Transmit 14/1  "Input current [mA]"
  Saturation2/1 -> Data Type Conversion17/1
  Data Type Conversion18/1 -> EtherCAT PDO Transmit 15/1  "Input current [mA]"
  Saturation3/1 -> Data Type Conversion18/1
  Data Type Conversion19/1 -> EtherCAT PDO Transmit 16/1  "Input current [mA]"
  Saturation4/1 -> Data Type Conversion19/1
  Data Type Conversion20/1 -> EtherCAT PDO Transmit 17/1  "Input current [mA]"
  Saturation5/1 -> Data Type Conversion20/1
  Bus Selector/2 -> Saturation1/1  "<signal2>"
  Bus Selector/3 -> Saturation2/1  "<signal3>"
  Bus Selector/4 -> Saturation3/1  "<signal4>"
  Bus Selector/5 -> Saturation4/1  "<signal5>"
  Bus Selector/6 -> Saturation5/1  "<signal6>"
  Bus Creator6/1 -> Angle [degrees]/1
  Demux/1 -> Bus Creator6/1
  Demux/2 -> Bus Creator6/2
  Demux/3 -> Bus Creator6/3
  Demux/4 -> Bus Creator6/4
  Demux/5 -> Bus Creator6/5
  Demux/6 -> Bus Creator6/6
  Demux1/2 -> Bus Creator7/2
  Demux1/3 -> Bus Creator7/3
  Demux1/1 -> Bus Creator7/1
  Demux1/6 -> Bus Creator7/6
  Bus Creator7/1 -> Actual current [mA]/1
  Data Type Conversion1/1 -> Demux1/1  "Actual current [mA]"
  Demux1/5 -> Bus Creator7/5
  Demux1/4 -> Bus Creator7/4
  Demux2/4 -> Bus Creator8/4
  Demux2/5 -> Bus Creator8/5
  Demux2/6 -> Bus Creator8/6
  Demux2/1 -> Bus Creator8/1
  Demux2/3 -> Bus Creator8/3
  Demux2/2 -> Bus Creator8/2
  Bus Creator8/1 -> Bus Creator9/4
  Bus Creator9/1 -> Status/1
  EtherCAT Async SDO Upload11/1 -> Bus Creator11/3
  EtherCAT Async SDO Upload6/1 -> Bus Creator10/1
  EtherCAT Async SDO Upload9/1 -> Bus Creator11/1
  EtherCAT Async SDO Upload8/1 -> Bus Creator10/3
  EtherCAT Async SDO Upload10/1 -> Bus Creator11/2
  EtherCAT Async SDO Upload7/1 -> Bus Creator10/2
  Constant2/1 -> EtherCAT Async SDO Upload8/1, EtherCAT Async SDO Upload7/1, EtherCAT Async SDO Upload6/1, EtherCAT Async SDO Upload11/1, EtherCAT Async SDO Upload10/1, EtherCAT Async SDO Upload9/1
  EtherCAT Async SDO Upload17/1 -> Bus Creator13/3
  EtherCAT Async SDO Upload12/1 -> Bus Creator12/1
  EtherCAT Async SDO Upload15/1 -> Bus Creator13/1
  EtherCAT Async SDO Upload14/1 -> Bus Creator12/3
  EtherCAT Async SDO Upload16/1 -> Bus Creator13/2
  EtherCAT Async SDO Upload13/1 -> Bus Creator12/2
  Constant3/1 -> EtherCAT Async SDO Upload14/1, EtherCAT Async SDO Upload13/1, EtherCAT Async SDO Upload12/1, EtherCAT Async SDO Upload17/1, EtherCAT Async SDO Upload16/1, EtherCAT Async SDO Upload15/1
  EtherCAT Async SDO Upload23/1 -> Bus Creator15/3
  EtherCAT Async SDO Upload18/1 -> Bus Creator14/1
  EtherCAT Async SDO Upload21/1 -> Bus Creator15/1
  EtherCAT Async SDO Upload20/1 -> Bus Creator14/3
  EtherCAT Async SDO Upload22/1 -> Bus Creator15/2
  EtherCAT Async SDO Upload19/1 -> Bus Creator14/2
  Constant4/1 -> EtherCAT Async SDO Upload20/1, EtherCAT Async SDO Upload19/1, EtherCAT Async SDO Upload18/1, EtherCAT Async SDO Upload23/1, EtherCAT Async SDO Upload22/1, EtherCAT Async SDO Upload21/1
  EtherCAT Async SDO Upload29/1 -> Bus Creator17/3
  EtherCAT Async SDO Upload24/1 -> Bus Creator16/1
  EtherCAT Async SDO Upload27/1 -> Bus Creator17/1
  EtherCAT Async SDO Upload26/1 -> Bus Creator16/3
  EtherCAT Async SDO Upload28/1 -> Bus Creator17/2
  EtherCAT Async SDO Upload25/1 -> Bus Creator16/2
  Constant5/1 -> EtherCAT Async SDO Upload26/1, EtherCAT Async SDO Upload25/1, EtherCAT Async SDO Upload24/1, EtherCAT Async SDO Upload29/1, EtherCAT Async SDO Upload28/1, EtherCAT Async SDO Upload27/1
  EtherCAT Async SDO Upload35/1 -> Bus Creator19/3
  EtherCAT Async SDO Upload30/1 -> Bus Creator18/1
  EtherCAT Async SDO Upload33/1 -> Bus Creator19/1
  EtherCAT Async SDO Upload32/1 -> Bus Creator18/3
  EtherCAT Async SDO Upload34/1 -> Bus Creator19/2
  EtherCAT Async SDO Upload31/1 -> Bus Creator18/2
  Constant6/1 -> EtherCAT Async SDO Upload32/1, EtherCAT Async SDO Upload31/1, EtherCAT Async SDO Upload30/1, EtherCAT Async SDO Upload35/1, EtherCAT Async SDO Upload34/1, EtherCAT Async SDO Upload33/1
  Bus Creator10/1 -> Bus Creator20/2
  Bus Creator11/1 -> Bus Creator21/2
  Bus Creator12/1 -> Bus Creator20/3
  Bus Creator13/1 -> Bus Creator21/3
  Bus Creator14/1 -> Bus Creator20/4
  Bus Creator15/1 -> Bus Creator21/4
  Bus Creator16/1 -> Bus Creator20/5
  Bus Creator17/1 -> Bus Creator21/5
  Bus Creator18/1 -> Bus Creator20/6
  Bus Creator19/1 -> Bus Creator21/6
  Bus Creator20/1 -> Bus Creator9/2
  Bus Creator21/1 -> Bus Creator9/3
  Extract Bits10/1 -> Data Type Conversion25/1  "ready to switch on"
  Extract Bits9/1 -> Data Type Conversion30/1  "limit  switch"
  Extract Bits17/1 -> Data Type Conversion27/1
  EtherCAT PDO Receive23/1 -> Extract Bits17/1, Extract Bits16/1
  Extract Bits14/1 -> Data Type Conversion21/1  "quick stop"
  Data Type Conversion28/1 -> Bus Creator26/2  "switch on disable"
  Data Type Conversion26/1 -> Bus Creator28/2  "STO selected"
  Data Type Conversion29/1 -> Extract Bits10/1, Extract Bits11/1, Extract Bits12/1, Extract Bits13/1, Extract Bits15/1, Extract Bits14/1
  EtherCAT PDO Receive22/1 -> Data Type Conversion29/1
  EtherCAT PDO Receive21/1 -> Extract Bits9/1  "Digital inputs []"
  Data Type Conversion21/1 -> ?  "quick stop"
  Extract Bits13/1 -> Data Type Conversion22/1  "fault"
  Extract Bits16/1 -> Data Type Conversion26/1  "STO selected"
  Extract Bits15/1 -> Data Type Conversion28/1  "switch on disable"
  Data Type Conversion22/1 -> Bus Creator25/2  "fault"
  Data Type Conversion25/1 -> Bus Creator2/2  "ready to switch on"
  Data Type Conversion27/1 -> ?  "HW enabled"
  Extract Bits11/1 -> Data Type Conversion24/1  "switched on"
  Data Type Conversion23/1 -> Bus Creator24/2  "operation enable"
  Data Type Conversion24/1 -> Bus Creator23/2  "switched on"
  Data Type Conversion30/1 -> Bus Creator27/2  "in limits"
  Extract Bits12/1 -> Data Type Conversion23/1  "operation enable"
  Extract Bits19/1 -> Data Type Conversion35/1  "ready to switch on"
  Extract Bits18/1 -> Data Type Conversion40/1  "limit  switch"
  Extract Bits26/1 -> Data Type Conversion37/1
  EtherCAT PDO Receive26/1 -> Extract Bits26/1, Extract Bits25/1
  Extract Bits23/1 -> Data Type Conversion31/1  "quick stop"
  Data Type Conversion38/1 -> Bus Creator26/3  "switch on disable"
  Data Type Conversion36/1 -> Bus Creator28/3  "STO selected"
  Data Type Conversion39/1 -> Extract Bits19/1, Extract Bits20/1, Extract Bits21/1, Extract Bits22/1, Extract Bits24/1, Extract Bits23/1
  EtherCAT PDO Receive25/1 -> Data Type Conversion39/1
  EtherCAT PDO Receive24/1 -> Extract Bits18/1  "Digital inputs []"
  Extract Bits22/1 -> Data Type Conversion32/1  "fault"
  Extract Bits25/1 -> Data Type Conversion36/1  "STO selected"
  Extract Bits24/1 -> Data Type Conversion38/1  "switch on disable"
  Data Type Conversion32/1 -> Bus Creator25/3  "fault"
  Data Type Conversion35/1 -> Bus Creator2/3  "ready to switch on"
  Data Type Conversion37/1 -> ?  "HW enabled"
  Extract Bits20/1 -> Data Type Conversion34/1  "switched on"
  Data Type Conversion33/1 -> Bus Creator24/3  "operation enable"
  Data Type Conversion34/1 -> Bus Creator23/3  "switched on"
  Data Type Conversion40/1 -> Bus Creator27/3  "in limits"
  Extract Bits21/1 -> Data Type Conversion33/1  "operation enable"
  Extract Bits28/1 -> Data Type Conversion45/1  "ready to switch on"
  Extract Bits27/1 -> Data Type Conversion50/1  "limit  switch"
  Extract Bits35/1 -> Data Type Conversion47/1
  EtherCAT PDO Receive29/1 -> Extract Bits35/1, Extract Bits34/1
  Extract Bits32/1 -> Data Type Conversion41/1  "quick stop"
  Data Type Conversion48/1 -> Bus Creator26/4  "switch on disable"
  Data Type Conversion46/1 -> Bus Creator28/4  "STO selected"
  Data Type Conversion49/1 -> Extract Bits28/1, Extract Bits29/1, Extract Bits30/1, Extract Bits31/1, Extract Bits33/1, Extract Bits32/1
  EtherCAT PDO Receive28/1 -> Data Type Conversion49/1
  EtherCAT PDO Receive27/1 -> Extract Bits27/1  "Digital inputs []"
  Extract Bits31/1 -> Data Type Conversion42/1  "fault"
  Extract Bits34/1 -> Data Type Conversion46/1  "STO selected"
  Extract Bits33/1 -> Data Type Conversion48/1  "switch on disable"
  Data Type Conversion42/1 -> Bus Creator25/4  "fault"
  Data Type Conversion45/1 -> Bus Creator2/4  "ready to switch on"
  Data Type Conversion47/1 -> ?  "HW enabled"
  Extract Bits29/1 -> Data Type Conversion44/1  "switched on"
  Data Type Conversion43/1 -> Bus Creator24/4  "operation enable"
  Data Type Conversion44/1 -> Bus Creator23/4  "switched on"
  Data Type Conversion50/1 -> Bus Creator27/4  "in limits"
  Extract Bits30/1 -> Data Type Conversion43/1  "operation enable"
  Extract Bits37/1 -> Data Type Conversion55/1  "ready to switch on"
  Extract Bits36/1 -> Data Type Conversion60/1  "limit  switch"
  Extract Bits44/1 -> Data Type Conversion57/1
  EtherCAT PDO Receive32/1 -> Extract Bits44/1, Extract Bits43/1
  Extract Bits41/1 -> Data Type Conversion51/1  "quick stop"
  Data Type Conversion58/1 -> Bus Creator26/5  "switch on disable"
  Data Type Conversion56/1 -> Bus Creator28/5  "STO selected"
  Data Type Conversion59/1 -> Extract Bits37/1, Extract Bits38/1, Extract Bits39/1, Extract Bits40/1, Extract Bits42/1, Extract Bits41/1
  EtherCAT PDO Receive31/1 -> Data Type Conversion59/1
  EtherCAT PDO Receive30/1 -> Extract Bits36/1  "Digital inputs []"
  Data Type Conversion51/1 -> ?  "quick stop"
  Extract Bits40/1 -> Data Type Conversion52/1  "fault"
  Extract Bits43/1 -> Data Type Conversion56/1  "STO selected"
  Extract Bits42/1 -> Data Type Conversion58/1  "switch on disable"
  Data Type Conversion52/1 -> Bus Creator25/5  "fault"
  Data Type Conversion55/1 -> Bus Creator2/5  "ready to switch on"
  Data Type Conversion57/1 -> ?  "HW enabled"
  Extract Bits38/1 -> Data Type Conversion54/1  "switched on"
  Data Type Conversion53/1 -> Bus Creator24/5  "operation enable"
  Data Type Conversion54/1 -> Bus Creator23/5  "switched on"
  Data Type Conversion60/1 -> Bus Creator27/5  "in limits"
  Extract Bits39/1 -> Data Type Conversion53/1  "operation enable"
  Extract Bits46/1 -> Data Type Conversion65/1  "ready to switch on"
  Extract Bits45/1 -> Data Type Conversion70/1  "limit  switch"
  Extract Bits53/1 -> Data Type Conversion67/1
  EtherCAT PDO Receive35/1 -> Extract Bits53/1, Extract Bits52/1
  Extract Bits50/1 -> Data Type Conversion61/1  "quick stop"
  Data Type Conversion68/1 -> Bus Creator26/6  "switch on disable"
  Data Type Conversion66/1 -> Bus Creator28/6  "STO selected"
  Data Type Conversion69/1 -> Extract Bits46/1, Extract Bits47/1, Extract Bits48/1, Extract Bits49/1, Extract Bits51/1, Extract Bits50/1
  EtherCAT PDO Receive34/1 -> Data Type Conversion69/1
  EtherCAT PDO Receive33/1 -> Extract Bits45/1  "Digital inputs []"
  Data Type Conversion61/1 -> ?  "quick stop"
  Extract Bits49/1 -> Data Type Conversion62/1  "fault"
  Extract Bits52/1 -> Data Type Conversion66/1  "STO selected"
  Extract Bits51/1 -> Data Type Conversion68/1  "switch on disable"
  Data Type Conversion62/1 -> Bus Creator25/6  "fault"
  Data Type Conversion65/1 -> Bus Creator2/6  "ready to switch on"
  Data Type Conversion67/1 -> ?  "HW enabled"
  Extract Bits47/1 -> Data Type Conversion64/1  "switched on"
  Data Type Conversion63/1 -> Bus Creator24/6  "operation enable"
  Data Type Conversion64/1 -> Bus Creator23/6  "switched on"
  Data Type Conversion70/1 -> Bus Creator27/6  "in limits"
  Extract Bits48/1 -> Data Type Conversion63/1  "operation enable"
  Bus Creator2/1 -> Bus Creator22/1  "Ready on"
  Bus Creator22/1 -> Bus Creator9/1
  Bus Creator23/1 -> Bus Creator22/2  "Drive on"
  Bus Creator24/1 -> Bus Creator22/3  "Drive active"
  Bus Creator25/1 -> Bus Creator22/4  "Fault"
  Data Type Conversion31/1 -> ?  "quick stop"
  Bus Creator26/1 -> Bus Creator22/5  "Switch on disabled"
  Bus Creator27/1 -> Bus Creator22/6  "Position in limits"
  Bus Creator28/1 -> Bus Creator22/7  "Emergency stop"
